simulink model "LKS_CarSim"  (Simulink 8.1)
settings: Solver=FixedStepDiscrete  StartTime=0.0  StopTime=500  FixedStep=0.001  RelTol=1e-3
PreLoadFcn:
  | load('Matrix.mat')
  | 
  | Vx = 100;
  | Q1 = 10;
  | Q2 = 5;
  | R = 25;
  | Ts = 0.01;
  | GearRatio = 17.25;
  | 
  | [K,Ad,Bd,Cd,Dd] = dLKS_LQR(Q1,Q2,R,Ts)
undefined symbols (not defined in the file or in its folder): Ad, fdesignblkfcn, gcbh, K
libraries: simulink x2, Solver_SF x1, dspadpt3 x1
settings Model: Creator=IVDL_Mola  LastModifiedBy=IVDL
settings DataIOCC: SignalLoggingSaveFormat=Dataset
settings OptimizationCC: ExpressionDepthLimit=128
settings DebuggingCC: FcnCallInpInsideContextMsg=EnableAllAsError  StateNameClashWarn=none
settings GRTTargetCC: CodeReplacementLibrary=None  CombineOutputUpdateFcns=on  CPPClassGenCompliant=on  GRTInterface=off

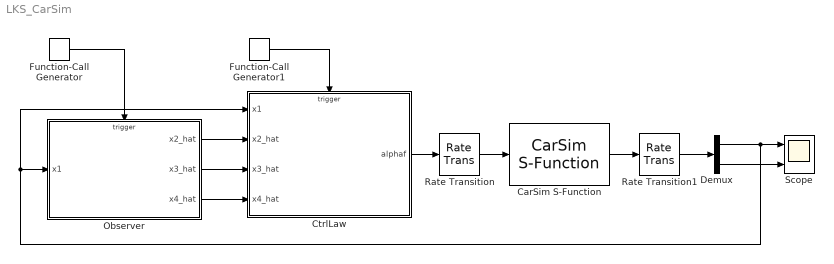
== system LKS_CarSim ==
  CarSim S-Function : Solver_SF/CarSim S-Function  Priority=1  VehicleCode=i_i  SIMFILE=simfile
  CtrlLaw : Subsystem
  Demux : Demux  Outputs=2
  Function-Call Generator : simulink/Ports & Subsystems/Function-Call Generator  sample_time=Ts  numberOfIterations=1
  Function-Call Generator1 : simulink/Ports & Subsystems/Function-Call Generator  sample_time=Ts  numberOfIterations=1
  Observer : Subsystem
  Rate Transition : RateTransition
  Rate Transition1 : RateTransition
  Scope : Scope  NumInputPorts=2
      settings: YMin=-1~-3  YMax=1~3
  wires:
  Observer/1(x2_hat) -> CtrlLaw/2(x2_hat)
  Observer/2(x3_hat) -> CtrlLaw/3(x3_hat)
  Observer/3(x4_hat) -> CtrlLaw/4(x4_hat)
  Function-Call Generator/1 -> Observer/Trigger
  Function-Call Generator1/1 -> CtrlLaw/Trigger
  CarSim S-Function/1 -> Rate Transition1/1
  CtrlLaw/1(alphaf) -> Rate Transition/1
  Rate Transition/1 -> CarSim S-Function/1
  Rate Transition1/1 -> Demux/1
  Demux/2 -> Scope/2
  Demux/1 -> CtrlLaw/1(x1), Observer/1(x1), Scope/1

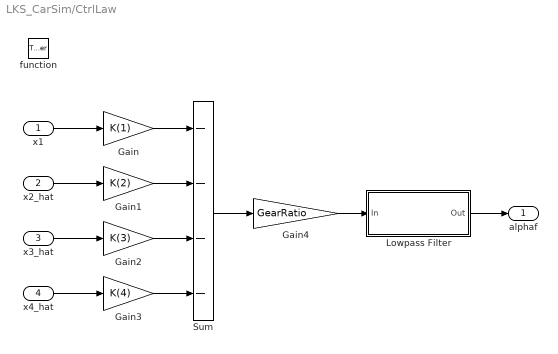
== system LKS_CarSim/CtrlLaw ==
  x1 : Inport
  x2_hat : Inport  Port=2
  x3_hat : Inport  Port=3
  x4_hat : Inport  Port=4
  function : TriggerPort  TriggerType=function-call  SampleTime=-1
  Gain : Gain  Gain=K(1)  OutDataTypeStr=double
  Gain1 : Gain  Gain=K(2)
  Gain2 : Gain  Gain=K(3)
  Gain3 : Gain  Gain=K(4)
  Gain4 : Gain  Gain=GearRatio  OutDataTypeStr=double
  Lowpass Filter : Subsystem  DialogController=fdesignblkfcn  DialogControllerArgs=DataTag1  InitFcn=fdesignblkfcn(gcbh, {'InitFcn'});  mask(Lowpass Filter){}
      mask help: Design a lowpass filter
      settings: CopyFcn=fdesignblkfcn(gcbh, {'CopyFcn'});
      mask Help: helpview(mapfilelocation('dsp'), 'dsplowpassfilter');
      mask Display: disp('Lowpass')
  Sum : Sum  Inputs=----  AccumDataTypeStr=double
  alphaf : Outport  OutDataTypeStr=double
  wires:
  x1/1 -> Gain/1
  Gain/1 -> Sum/1
  Gain1/1 -> Sum/2
  Gain3/1 -> Sum/4
  Gain2/1 -> Sum/3
  Sum/1 -> Gain4/1
  x2_hat/1 -> Gain1/1
  x3_hat/1 -> Gain2/1
  x4_hat/1 -> Gain3/1
  Gain4/1 -> Lowpass Filter/1(In)
  Lowpass Filter/1(Out) -> alphaf/1

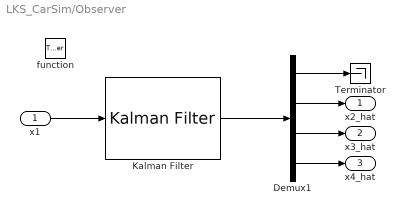
== system LKS_CarSim/Observer ==
  x1 : Inport
  function : TriggerPort  TriggerType=function-call  SampleTime=-1
  Demux1 : Demux
  Kalman Filter : dspadpt3/Kalman Filter  num_targets=1  sourceEnable=Always  isReset=on  X=zeros([4, 1])  P=10*eye(4)  A=Ad  sourceMeasure=Specify via Dialog  H=Cd  Q=0.05*eye(4)  R=eye(1)  isOutputEstMeasure=off  isOutputEstState=on  isOutputEstError=off  isOutputPrdMeasure=off  isOutputPrdState=off  isOutputPrdError=off
  Terminator : Terminator
  x2_hat : Outport
  x3_hat : Outport  Port=2
  x4_hat : Outport  Port=3
  wires:
  Demux1/3 -> x3_hat/1
  Demux1/1 -> Terminator/1
  Kalman Filter/1 -> Demux1/1
  x1/1 -> Kalman Filter/1
  Demux1/2 -> x2_hat/1
  Demux1/4 -> x4_hat/1

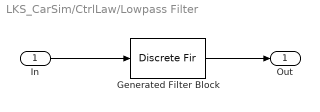
== system LKS_CarSim/CtrlLaw/Lowpass Filter ==
  In : Inport
  Generated Filter Block : DiscreteFir  Tag=BlockMethodSubSystem  Coefficients=[-0.12703898269324654 0.60128910085241971 0.60128910085241971 -0.12703898269324654]  InputProcessing=Columns as channels (frame based)
  Out : Outport
  wires:
  In/1 -> Generated Filter Block/1
  Generated Filter Block/1 -> Out/1
